simulink model "Scenario_TJunction_noTrafficLights_older"  (R2021a)
settings: Solver=VariableStepAuto  StartTime=0.0  StopTime=10.0  RelTol=1e-3
model workspace (MAT data in the model file):
  Kz_dif = Simulink.Parameter
  Kz_dif.Value = Simulink.data.Expression
  Kz_dif.Value.ExpressionString = " L_dif / (Lc + ds)"
  Kz_dif.DataType = 'auto'
  Kz_dif.Dimensions = -1
  Kz_il = Simulink.Parameter
  Kz_il.Value = Simulink.data.Expression
  Kz_il.Value.ExpressionString = " L_il / (Lc + ds)"
  Kz_il.DataType = 'auto'
  Kz_il.Dimensions = -1
  Kz_ir = Simulink.Parameter
  Kz_ir.Value = Simulink.data.Expression
  Kz_ir.Value.ExpressionString = " L_ir / (Lc + ds)"
  Kz_ir.DataType = 'auto'
  Kz_ir.Dimensions = -1
  Kz_is = Simulink.Parameter
  Kz_is.Value = Simulink.data.Expression
  Kz_is.Value.ExpressionString = " L_is / (Lc + ds)"
  Kz_is.DataType = 'auto'
  Kz_is.Dimensions = -1
  Kz_long = Simulink.Parameter
  Kz_long.Value = Simulink.data.Expression
  Kz_long.Value.ExpressionString = " L_long / (Lc + ds)"
  Kz_long.Description = 'Segmentkapazität (wie viele autos passen hinein)'
  Kz_long.DataType = 'auto'
  Kz_long.Dimensions = -1
  Kz_pre = Simulink.Parameter
  Kz_pre.Value = Simulink.data.Expression
  Kz_pre.Value.ExpressionString = " L_pre / (Lc + ds)"
  Kz_pre.DataType = 'auto'
  Kz_pre.Dimensions = -1
  L_dif = Simulink.Parameter
  L_dif.Value = Simulink.data.Expression
  L_dif.Value.ExpressionString = "L_long-L_pre"
  L_dif.Description = 'Differenz zwischen Abbiegerspurlänge und normaler straßenlänge'
  L_dif.DataType = 'auto'
  L_dif.Dimensions = -1
  L_il = Simulink.Parameter
  L_il.Value = 30
  L_il.Description = 'Länge der innenkreuzungssegments, das linksabbieger durchqueren'
  L_il.DataType = 'auto'
  L_il.Dimensions = [1 1]
  L_ir = Simulink.Parameter
  L_ir.Value = 23
  L_ir.Description = 'Länge der innenkreuzungssegments, das rechtsabbieger durchqueren'
  L_ir.DataType = 'auto'
  L_ir.Dimensions = [1 1]
  L_is = Simulink.Parameter
  L_is.Value = 35
  L_is.Description = 'Länge der innenkreuzungssegments, das geradeausfahrer durchqueren'
  L_is.DataType = 'auto'
  L_is.Dimensions = [1 1]
  L_long = Simulink.Parameter
  L_long.Value = 52.8
  L_long.Description = 'Langes straßensegment  (52.8 meter)'
  L_long.DataType = 'auto'
  L_long.Dimensions = [1 1]
  L_pre = Simulink.Parameter
  L_pre.Value = 20
  L_pre.Description = 'Länge der Abbiegespuren'
  L_pre.DataType = 'auto'
  L_pre.Dimensions = [1 1]
  Lc = Simulink.Parameter
  Lc.Value = 4.4
  Lc.Description = 'Länge eines autos'
  Lc.DataType = 'auto'
  Lc.Dimensions = [1 1]
  Rk = Simulink.Parameter
  Rk.Value = Simulink.data.Expression
  Rk.Value.ExpressionString = " Lc / v"
  Rk.Description = 'Flussrate zwischen den Kanten (bei speed v)'
  Rk.DataType = 'auto'
  Rk.Dimensions = -1
  Tz_dif = Simulink.Parameter
  Tz_dif.Value = Simulink.data.Expression
  Tz_dif.Value.ExpressionString = " L_dif / v"
  Tz_dif.DataType = 'auto'
  Tz_dif.Dimensions = -1
  Tz_il = Simulink.Parameter
  Tz_il.Value = Simulink.data.Expression
  Tz_il.Value.ExpressionString = " L_il / v"
  Tz_il.DataType = 'auto'
  Tz_il.Dimensions = -1
  Tz_ir = Simulink.Parameter
  Tz_ir.Value = Simulink.data.Expression
  Tz_ir.Value.ExpressionString = " L_ir / v"
  Tz_ir.DataType = 'auto'
  Tz_ir.Dimensions = -1
  Tz_is = Simulink.Parameter
  Tz_is.Value = Simulink.data.Expression
  Tz_is.Value.ExpressionString = " L_is / v"
  Tz_is.DataType = 'auto'
  Tz_is.Dimensions = -1
  Tz_long = Simulink.Parameter
  Tz_long.Value = Simulink.data.Expression
  Tz_long.Value.ExpressionString = " L_long / v"
  Tz_long.Description = 'Segment durchfahrtzeit: wie lange würde ein auto brauchen,um
    | ungehindert durch das segment zu fahren.'
  Tz_long.DataType = 'auto'
  Tz_long.Dimensions = -1
  Tz_pre = Simulink.Parameter
  Tz_pre.Value = Simulink.data.Expression
  Tz_pre.Value.ExpressionString = " L_pre / v"
  Tz_pre.DataType = 'auto'
  Tz_pre.Dimensions = -1
  ds = Simulink.Parameter
  ds.Value = Simulink.data.Expression
  ds.Value.ExpressionString = "v*dt"
  ds.DataType = 'auto'
  ds.Dimensions = -1
  dt = Simulink.Parameter
  dt.Value = 1
  dt.Description = 'temporaler sicherheitsabstand'
  dt.DataType = 'auto'
  dt.Dimensions = [1 1]
  v = Simulink.Parameter
  v.Value = 13.89
  v.Description = 'geschwindigkeit eines autos
    | (km/h : 3.75 = m/s)
    | 	30km/h = 8,34m/s
    | 	20km/h = 5.56m/s
    | 	50km/h = 13.89m/s
    | '
  v.DataType = 'auto'
  v.Dimensions = [1 1]
libraries: EdgesLibrary x26, StreetLanesLibrary x24, SourcesAndSinksLibrary x6
settings Model: Creator=phill  LastModifiedBy=phill
settings SolverCC: ZeroCrossAlgorithm=Adaptive

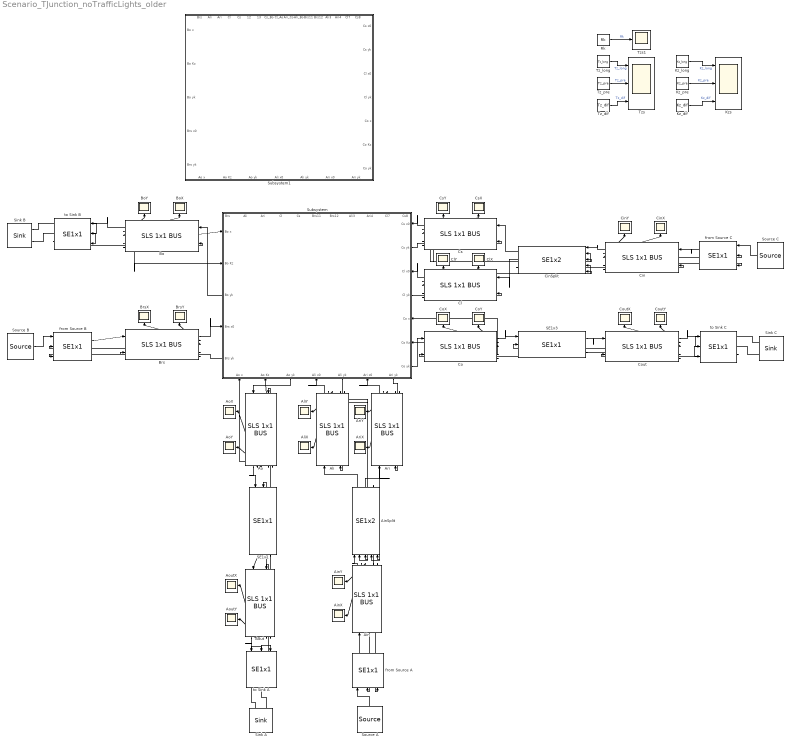
== system Scenario_TJunction_noTrafficLights_older ==
  Ain : StreetLanesLibrary/SLS 1x1 BUS  Kz=Kz_dif  Tz=Tz_dif
  AinSplit : EdgesLibrary/SE1x2  Rk1=0.5*Rk  Rk2=0.5*Rk
  AinX : Scope
  AinY : Scope
  Ali : StreetLanesLibrary/SLS 1x1 BUS  Kz=Kz_pre  Tz=Tz_pre
  AliX : Scope
  AliY : Scope
  Ao : StreetLanesLibrary/SLS 1x1 BUS  Kz=Kz_pre  Tz=Tz_pre
  AoX : Scope
  AoY : Scope
  Aout : StreetLanesLibrary/SLS 1x1 BUS  Kz=Kz_dif  Tz=Tz_dif
  AoutX : Scope
  AoutY : Scope
  Ari : StreetLanesLibrary/SLS 1x1 BUS  Kz=Kz_pre  Tz=Tz_pre
  AriX : Scope
  AriY : Scope
  Bo : StreetLanesLibrary/SLS 1x1 BUS  Kz=Kz_pre  Tz=Tz_pre
  BoX : Scope
  BoY : Scope
  Brs : StreetLanesLibrary/SLS 1x1 BUS  Kz=Kz_pre  Tz=Tz_pre
  BrsX : Scope
  BrsY : Scope
  Cin : StreetLanesLibrary/SLS 1x1 BUS  Kz=Kz_dif  Tz=Tz_dif
  CinSplit : EdgesLibrary/SE1x2  Rk1=0.5*Rk  Rk2=0.5*Rk
  CinX : Scope
  CinY : Scope
  Cl : StreetLanesLibrary/SLS 1x1 BUS  Kz=Kz_pre  Tz=Tz_pre
  ClX : Scope
  ClY : Scope
  Co : StreetLanesLibrary/SLS 1x1 BUS  Kz=Kz_pre  Tz=Tz_pre
  CoX : Scope
  CoY : Scope
  Cout : StreetLanesLibrary/SLS 1x1 BUS  Kz=Kz_dif  Tz=Tz_dif
  CoutX : Scope
  CoutY : Scope
  Cs : StreetLanesLibrary/SLS 1x1 BUS  Kz=Kz_pre  Tz=Tz_pre
  CsX : Scope
  CsY : Scope
  Kz_dif : Constant  Value=Kz_dif
  Kz_long : Constant  Value=Kz_long
  Kz_pre : Constant  Value=Kz_pre
  Kzs : Scope  NumInputPorts=3
  Rk : Constant  Value=Rk
  SE1x1 : EdgesLibrary/SE1x1  Rk=Rk
  SE1x3 : EdgesLibrary/SE1x1  Rk=Rk
  Sink A : SourcesAndSinksLibrary/Sink  SystemSampleTime=-1  VariantActivationTime=update diagram  Latency=0  AutoFrameSizeCalculation=off
      settings: PortSchema="{\"entries\":[{\"content\":{\"sides\":[{\"content\":{\"connectorIds\":[\"Out1\",\"Out2\"]},\"type\":\"ConnectorPlacement.EquallySpacedRectSide\",\"uuid\":\"9fd2383e-3590-4f0f-bafc-5a4adfbb32b4\"},{\"content\":{\"connectorIds\":[],\"side\":\"RIGHT\"},\"type\":\"ConnectorPlacement.EquallySpacedRectSide\",\"uuid\":\"1e687aa9-1098-45bd-a1f6-ea403f3f2897\"},{\"content\":{\"connectorIds\":[],\"side\":\"TOP\"},\"type\":\"ConnectorPlacement.EquallySpacedRectSide\",\"uuid\":\"fe6eaa71-085c-414b-983a-a0e72e52a49c\"}]},\"type\":\"ConnectorPlacement.EquallySpacedConnector\",\"uuid\":\"370c1712-4373-4726-99c2-6cb04807ece1\"}],\"packageUris\":[\"http://schema.mathworks.com/mf0/Connector/R2020b\"],\"version\":\"1.0\"}"
  Sink B : SourcesAndSinksLibrary/Sink  SystemSampleTime=-1  VariantActivationTime=update diagram  Latency=0  AutoFrameSizeCalculation=off
      settings: PortSchema="{\"entries\":[{\"content\":{\"sides\":[{\"content\":{\"connectorIds\":[\"Out1\",\"Out2\"]},\"type\":\"ConnectorPlacement.EquallySpacedRectSide\",\"uuid\":\"9fd2383e-3590-4f0f-bafc-5a4adfbb32b4\"},{\"content\":{\"connectorIds\":[],\"side\":\"RIGHT\"},\"type\":\"ConnectorPlacement.EquallySpacedRectSide\",\"uuid\":\"1e687aa9-1098-45bd-a1f6-ea403f3f2897\"},{\"content\":{\"connectorIds\":[],\"side\":\"TOP\"},\"type\":\"ConnectorPlacement.EquallySpacedRectSide\",\"uuid\":\"fe6eaa71-085c-414b-983a-a0e72e52a49c\"}]},\"type\":\"ConnectorPlacement.EquallySpacedConnector\",\"uuid\":\"370c1712-4373-4726-99c2-6cb04807ece1\"}],\"packageUris\":[\"http://schema.mathworks.com/mf0/Connector/R2020b\"],\"version\":\"1.0\"}"
  Sink C : SourcesAndSinksLibrary/Sink  SystemSampleTime=-1  VariantActivationTime=update diagram  Latency=0  AutoFrameSizeCalculation=off
      settings: PortSchema="{\"entries\":[{\"content\":{\"sides\":[{\"content\":{\"connectorIds\":[\"Out1\",\"Out2\"]},\"type\":\"ConnectorPlacement.EquallySpacedRectSide\",\"uuid\":\"9fd2383e-3590-4f0f-bafc-5a4adfbb32b4\"},{\"content\":{\"connectorIds\":[],\"side\":\"RIGHT\"},\"type\":\"ConnectorPlacement.EquallySpacedRectSide\",\"uuid\":\"1e687aa9-1098-45bd-a1f6-ea403f3f2897\"},{\"content\":{\"connectorIds\":[],\"side\":\"TOP\"},\"type\":\"ConnectorPlacement.EquallySpacedRectSide\",\"uuid\":\"fe6eaa71-085c-414b-983a-a0e72e52a49c\"}]},\"type\":\"ConnectorPlacement.EquallySpacedConnector\",\"uuid\":\"370c1712-4373-4726-99c2-6cb04807ece1\"}],\"packageUris\":[\"http://schema.mathworks.com/mf0/Connector/R2020b\"],\"version\":\"1.0\"}"
  Source A : SourcesAndSinksLibrary/Source  SystemSampleTime=-1  VariantActivationTime=update diagram  Latency=0  AutoFrameSizeCalculation=off
  Source B : SourcesAndSinksLibrary/Source  SystemSampleTime=-1  VariantActivationTime=update diagram  Latency=0  AutoFrameSizeCalculation=off
  Source C : SourcesAndSinksLibrary/Source  SystemSampleTime=-1  VariantActivationTime=update diagram  Latency=0  AutoFrameSizeCalculation=off
  Subsystem : Subsystem  mask{Kz_left=Kz_il, Tz_left=Tz_il, Kz_straight=Kz_is, Tz_straight=Tz_is, Kz_right=Kz_ir, Tz_right=Tz_ir, Rk=Rk}
      settings: PortSchema="{\"entries\":[{\"content\":{\"sides\":[{\"content\":{\"connectorIds\":[\"In1\",\"In2\",\"Out12\",\"In3\",\"Out13\"]},\"type\":\"ConnectorPlacement.EquallySpacedRectSide\",\"uuid\":\"e697a1b6-0b61-4022-ac11-26e96db57f42\"},{\"content\":{\"connectorIds\":[\"In14\",\"Out1\",\"In15\",\"Out2\",\"In16\",\"In17\",\"Out3\"],\"side\":\"RIGHT\"},\"type\":\"ConnectorPlacement.EquallySpacedRectSide\",\"uuid\":\"73d64b2d-08c1-4421-9fcb-daf7d69c3a51\"},{\"content\":{\"connectorIds\":[\"Out7\",\"Out8\",\"Out9\",\"Out10\",\"Out11\",\"In4\",\"In5\",\"In6\",\"In7\",\"In8\",\"In9\"],\"side\":\"TOP\"},\"type\":\"ConnectorPlacement.EquallySpacedRectSide\",\"uuid\":\"d1fda098-bb61-48fd-b619-252fd8b1727b\"},{\"content\":{\"connectorIds\":[\"In10\",\"In11\",\"Out4\",\"In12\",\"Out5\",\"In13\",\"Out6\"],\"side\":\"BOTTOM\"},\"type\":\"ConnectorPlacement.EquallySpacedRectSide\",\"uuid\":\"eb83420e-ae17-428e-89d3-8e583c14dd5f\"}]},\"type\":\"ConnectorPlacement.EquallySpacedConnector\",\"uuid\":\"f702b239-8bcf-4357-be27-0d0ceba5c268\"}],\"packageUris\":[\"http://schema.mathworks.com/mf0/Connector/R2020b\"],\"version\":\"1.0\"}"
      mask Display:
      | %image('$imagefile'); % Use "Edit Image" on toolstrip to change.
      | disp('T \n\n');
      | KzS = get_param(gcb,'Kz_straight');
      | TzS = get_param(gcb,'Tz_straight');
      | KzR = get_param(gcb,'Kz_right');
      | TzR = get_param(gcb,'Tz_right');
      | KzL = get_param(gcb,'Kz_left');
      | TzL = get_param(gcb,'Tz_left');
      | Rk = get_param(gcb,'Rk');
      | disp(['Rk = ', Rk, ' | Kz/Tz L = ', KzL, ' ', TzL, ' | Kz/Tz S = ', KzS, ' ', TzS, ' | Kz/Tz R = ', KzR, ' ', TzR]);
  Subsystem1 : Subsystem  mask{Kz_left=0, Tz_left=0, Kz_straight=0, Tz_straight=0, Kz_right=0, Tz_right=0, Rk=0}
      settings: PortSchema="{\"entries\":[{\"content\":{\"sides\":[{\"content\":{\"connectorIds\":[\"In1\",\"In2\",\"Out18\",\"In3\",\"Out19\"]},\"type\":\"ConnectorPlacement.EquallySpacedRectSide\",\"uuid\":\"96c9f498-b0bc-4839-a476-8992d885d35a\"},{\"content\":{\"connectorIds\":[\"In14\",\"Out1\",\"In15\",\"Out2\",\"In16\",\"In17\",\"Out3\"],\"side\":\"RIGHT\"},\"type\":\"ConnectorPlacement.EquallySpacedRectSide\",\"uuid\":\"11ab0cdd-7db6-4f39-a252-8216aa6322d2\"},{\"content\":{\"connectorIds\":[\"Out7\",\"Out8\",\"Out9\",\"Out10\",\"Out11\",\"Out12\",\"Out13\",\"Out14\",\"Out15\",\"Out16\",\"Out17\",\"In4\",\"In5\",\"In6\",\"In7\",\"In8\",\"In9\"],\"side\":\"TOP\"},\"type\":\"ConnectorPlacement.EquallySpacedRectSide\",\"uuid\":\"f8ff7b80-df82-4633-b83a-80e44c4409b9\"},{\"content\":{\"connectorIds\":[\"In10\",\"In11\",\"Out4\",\"In12\",\"Out5\",\"In13\",\"Out6\"],\"side\":\"BOTTOM\"},\"type\":\"ConnectorPlacement.EquallySpacedRectSide\",\"uuid\":\"816219a6-152c-447e-807e-ad4d62c96b47\"}]},\"type\":\"ConnectorPlacement.EquallySpacedConnector\",\"uuid\":\"16c591aa-9a6b-4cb9-9c60-a78ca06e8a6b\"}],\"packageUris\":[\"http://schema.mathworks.com/mf0/Connector/R2020b\"],\"version\":\"1.0\"}"
      mask Display:
      | %image('$imagefile'); % Use "Edit Image" on toolstrip to change.
      | disp('T \n\n');
      | KzS = get_param(gcb,'Kz_straight');
      | TzS = get_param(gcb,'Tz_straight');
      | KzR = get_param(gcb,'Kz_right');
      | TzR = get_param(gcb,'Tz_right');
      | KzL = get_param(gcb,'Kz_left');
      | TzL = get_param(gcb,'Tz_left');
      | Rk = get_param(gcb,'Rk');
      | disp(['Rk = ', Rk, ' | Kz/Tz L = ', KzL, ' ', TzL, ' | Kz/Tz S = ', KzS, ' ', TzS, ' | Kz/Tz R = ', KzR, ' ', TzR]);
  Tz_dif : Constant  Value=Tz_dif
  Tz_long : Constant  Value=Tz_long
  Tz_pre : Constant  Value=Tz_pre
  Tzs : Scope  NumInputPorts=3
  Tzs1 : Scope
  from Source A : EdgesLibrary/SE1x1  Rk=Rk
  from Source B : EdgesLibrary/SE1x1  Rk=Rk
  from Source C : EdgesLibrary/SE1x1  Rk=Rk
  to Sink A : EdgesLibrary/SE1x1  Rk=Rk
  to Sink B : EdgesLibrary/SE1x1  Rk=Rk
  to Sink C : EdgesLibrary/SE1x1  Rk=Rk
  wires:
  Ao/6 -> Subsystem/10(Ao x)
  Ao/7 -> Subsystem/11(Ao Kz)
  Subsystem/4(Ao yk) -> Ao/1
  Ali/2 -> Subsystem/12(Ali x0)
  Subsystem/5(Ali yk) -> Ali/2
  Ari/2 -> Subsystem/13(Ari x0)
  Subsystem/6(Ari yk) -> Ari/2
  AinSplit/2 -> Ari/1
  Ari/7 -> AinSplit/5
  Ari/6 -> AinSplit/4
  AinSplit/1 -> Ali/1
  Ali/7 -> AinSplit/3
  Ali/6 -> AinSplit/2
  Ao/2 -> SE1x1/1
  SE1x1/2 -> Ao/2
  Ain/2 -> AinSplit/1
  AinSplit/3 -> Ain/2
  Aout/6 -> SE1x1/2
  Aout/7 -> SE1x1/3
  SE1x1/1 -> Aout/1
  Source A/1 -> from Source A/1
  from Source A/1 -> Ain/1
  Ain/7 -> from Source A/3
  Ain/6 -> from Source A/2
  to Sink A/2 -> Aout/2
  Aout/2 -> to Sink A/1
  Sink A/1 -> to Sink A/2
  Sink A/2 -> to Sink A/3
  Co/6 -> Subsystem/16(Co x)
  Co/7 -> Subsystem/17(Co Kz)
  Subsystem/3(Co yk) -> Co/1
  Subsystem/2(Cl yk) -> Cl/2
  Cl/2 -> Subsystem/15(Cl x0)
  Subsystem/1(Cs yk) -> Cs/2
  Cs/2 -> Subsystem/14(Cs x0)
  Bo/6 -> Subsystem/1(Bo x)
  Bo/7 -> Subsystem/2(Bo Kz)
  Subsystem/12(Bo yk) -> Bo/1
  Brs/2 -> Subsystem/3(Brs x0)
  Subsystem/13(Brs yk) -> Brs/2
  SE1x3/2 -> Co/2
  Co/2 -> SE1x3/1
  SE1x3/1 -> Cout/1
  Cout/7 -> SE1x3/3
  Cout/6 -> SE1x3/2
  Cs/6 -> CinSplit/2
  Cs/7 -> CinSplit/3
  CinSplit/1 -> Cs/1
  Cl/6 -> CinSplit/4
  Cl/7 -> CinSplit/5
  CinSplit/2 -> Cl/1
  CinSplit/3 -> Cin/2
  Cin/2 -> CinSplit/1
  Sink C/1 -> to Sink C/2
  Sink C/2 -> to Sink C/3
  Cout/2 -> to Sink C/1
  to Sink C/2 -> Cout/2
  Source C/1 -> from Source C/1
  Cin/6 -> from Source C/2
  Cin/7 -> from Source C/3
  from Source C/1 -> Cin/1
  Source B/1 -> from Source B/1
  Sink B/2 -> to Sink B/3
  Sink B/1 -> to Sink B/2
  Bo/2 -> to Sink B/1
  to Sink B/2 -> Bo/2
  Brs/6 -> from Source B/2
  Brs/7 -> from Source B/3
  from Source B/1 -> Brs/1
  Bo/4 -> BoY/1
  Cs/4 -> CsY/1
  Cl/4 -> ClY/1
  Cl/3 -> ClX/1
  Co/3 -> CoX/1
  Co/4 -> CoY/1
  Cs/3 -> CsX/1
  Brs/3 -> BrsX/1
  Brs/4 -> BrsY/1
  Bo/3 -> BoX/1
  Cin/4 -> CinY/1
  Cin/3 -> CinX/1
  Cout/3 -> CoutX/1
  Cout/4 -> CoutY/1
  Ao/3 -> AoX/1
  Ao/4 -> AoY/1
  Ali/4 -> AliY/1
  Ali/3 -> AliX/1
  Ari/4 -> AriY/1
  Ari/3 -> AriX/1
  Aout/3 -> AoutX/1
  Aout/4 -> AoutY/1
  Ain/4 -> AinY/1
  Ain/3 -> AinX/1
  Tz_long/1 -> Tzs/1  "Tz_long"
  Tz_pre/1 -> Tzs/2  "Tz_pre"
  Tz_dif/1 -> Tzs/3  "Tz_dif"
  Kz_long/1 -> Kzs/1  "Kz_long"
  Kz_pre/1 -> Kzs/2  "Kz_pre"
  Kz_dif/1 -> Kzs/3  "Kz_dif"
  Rk/1 -> Tzs1/1  "Rk"

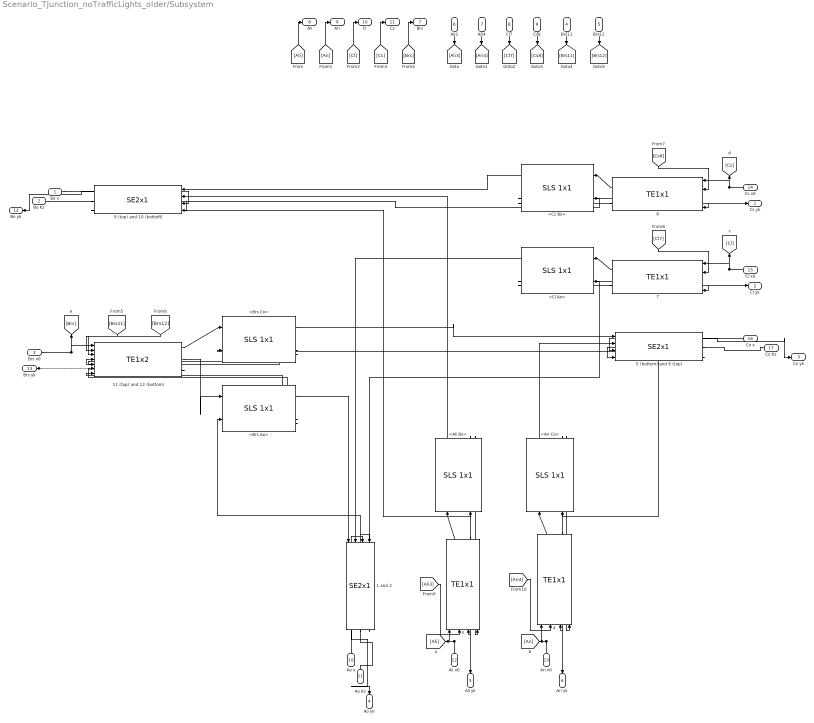
== system Scenario_TJunction_noTrafficLights_older/Subsystem ==
  Bo x : Inport
  Bo Kz : Inport  Port=2
  Brs x0 : Inport  Port=3
  Brs11 : Inport  Port=4
  Brs12 : Inport  Port=5
  Ali3 : Inport  Port=6
  Ari4 : Inport  Port=7
  Cl7 : Inport  Port=8
  Cs8 : Inport  Port=9
  Ao x : Inport  Port=10
  Ao Kz : Inport  Port=11
  Ali x0 : Inport  Port=12
  Ari x0 : Inport  Port=13
  Cs x0 : Inport  Port=14
  Cl x0 : Inport  Port=15
  Co x : Inport  Port=16
  Co Kz : Inport  Port=17
  1 and 2 : EdgesLibrary/SE2x1  Rk1=Rk  Rk2=Rk
  11 (top) and 12 (bottom) : EdgesLibrary/TE1x2  Rk1=0.5*Rk  Rk2=0.5*Rk
  {3..4,7..8} (4 alike) : EdgesLibrary/TE1x1  Rk=Rk
  5 (bottom) and 6 (top) : EdgesLibrary/SE2x1  Rk1=Rk  Rk2=Rk
  9 (top) and 10 (bottoM) : EdgesLibrary/SE2x1  Rk1=Rk  Rk2=Rk
  <Ali Bo> : StreetLanesLibrary/SLS 1x1  Kz=Kz_left  Tz=Tz_left
  <Ari Co> : StreetLanesLibrary/SLS 1x1  Kz=Kz_right  Tz=Tz_right
  <Brs Ao> : StreetLanesLibrary/SLS 1x1  Kz=Kz_right  Tz=Tz_right
  <Brs Co> : StreetLanesLibrary/SLS 1x1  Kz=Kz_straight  Tz=Tz_straight
  <Cl Ao> : StreetLanesLibrary/SLS 1x1  Kz=Kz_left  Tz=Tz_left
  <Cs Bo> : StreetLanesLibrary/SLS 1x1  Kz=Kz_straight  Tz=Tz_straight
  Cs yk : Outport
  Cl yk : Outport  Port=2
  Co yk : Outport  Port=3
  Ao yk : Outport  Port=4
  Ali yk : Outport  Port=5
  Ari yk : Outport  Port=6
  Brs : Outport  Port=7
  Ali : Outport  Port=8
  Ari : Outport  Port=9
  Cl : Outport  Port=10
  Cs : Outport  Port=11
  Bo yk : Outport  Port=12
  Brs yk : Outport  Port=13
  wires:
  11 (top) and 12 (bottom)/2 -> <Brs Ao>/1
  11 (top) and 12 (bottom)/3 -> Brs yk/1
  3/2 -> Ali yk/1
  3/1 -> <Ali Bo>/1
  Ari x0/1 -> [Ari], 4/1
  <Cs Bo>/2 -> 9 (top) and 10 (bottoM)/1
  <Cs Bo>/8 -> 8/4
  <Cl Ao>/8 -> 7/4
  Co x/1 -> 5 (bottom) and 6 (top)/3
  5 (bottom) and 6 (top)/1 -> Co yk/1
  5 (bottom) and 6 (top)/3 -> <Ari Co>/2
  <Ari Co>/8 -> 4/4
  <Ali Bo>/8 -> 3/4
  Ao x/1 -> 1 and 2/3
  Brs x0/1 -> 11 (top) and 12 (bottom)/1, [Brs]
  <Brs Co>/2 -> 5 (bottom) and 6 (top)/1
  <Cl Ao>/7 -> 7/3
  <Cl Ao>/2 -> 1 and 2/2
  9 (top) and 10 (bottoM)/2 -> <Cs Bo>/2
  [Brs] -> Brs/1
  <Ari Co>/2 -> 5 (bottom) and 6 (top)/2
  7/1 -> <Cl Ao>/1
  Cl x0/1 -> [Cl], 7/1
  4/1 -> <Ari Co>/1
  <Ari Co>/7 -> 4/3
  <Brs Ao>/2 -> 1 and 2/1
  Ao Kz/1 -> 1 and 2/4
  <Brs Ao>/7 -> 11 (top) and 12 (bottom)/6
  <Brs Ao>/8 -> 11 (top) and 12 (bottom)/7
  Co Kz/1 -> 5 (bottom) and 6 (top)/4
  8/2 -> Cs yk/1
  Bo Kz/1 -> 9 (top) and 10 (bottoM)/4
  1 and 2/3 -> <Cl Ao>/2
  <Brs Co>/8 -> 11 (top) and 12 (bottom)/5
  [Brs12] -> 11 (top) and 12 (bottom)/3
  9 (top) and 10 (bottoM)/3 -> <Ali Bo>/2
  <Ali Bo>/7 -> 3/3
  1 and 2/2 -> <Brs Ao>/2
  Ali x0/1 -> [Ali], 3/1
  <Brs Co>/7 -> 11 (top) and 12 (bottom)/4
  1 and 2/1 -> Ao yk/1
  <Ali Bo>/2 -> 9 (top) and 10 (bottoM)/2
  [Ari4] -> 4/2
  5 (bottom) and 6 (top)/2 -> <Brs Co>/2
  8/1 -> <Cs Bo>/1
  4/2 -> Ari yk/1
  <Cs Bo>/7 -> 8/3
  Cs x0/1 -> [Cs], 8/1
  [Ali3] -> 3/2
  [Brs11] -> 11 (top) and 12 (bottom)/2
  11 (top) and 12 (bottom)/1 -> <Brs Co>/1
  Bo x/1 -> 9 (top) and 10 (bottoM)/3
  [Cl7] -> 7/2
  9 (top) and 10 (bottoM)/1 -> Bo yk/1
  [Ari] -> Ari/1
  [Ali] -> Ali/1
  7/2 -> Cl yk/1
  [Cs8] -> 8/2
  [Cl] -> Cl/1
  [Cs] -> Cs/1
  Ali3/1 -> [Ali3]
  Ari4/1 -> [Ari4]
  Cl7/1 -> [Cl7]
  Cs8/1 -> [Cs8]
  Brs11/1 -> [Brs11]
  Brs12/1 -> [Brs12]

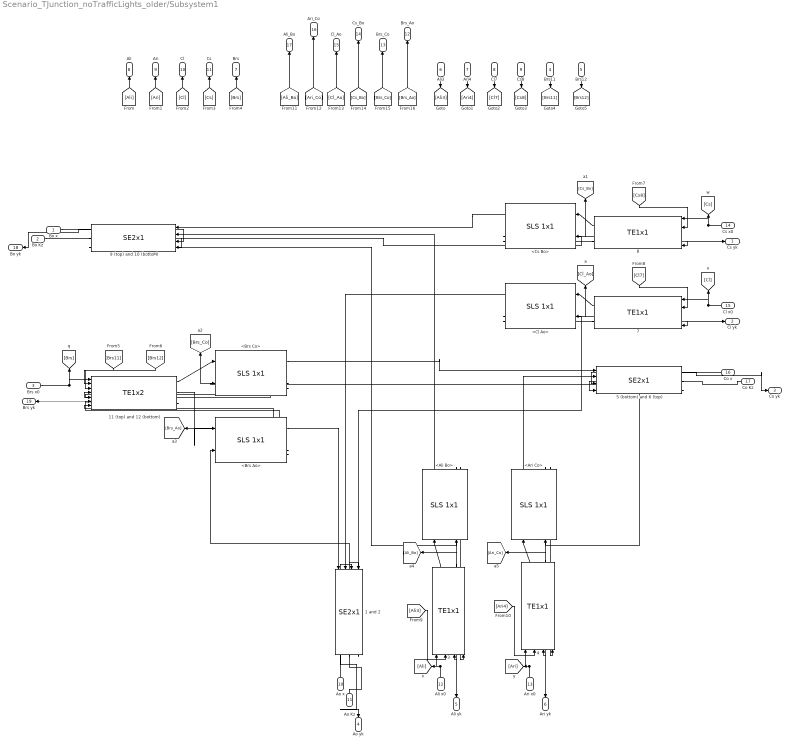
== system Scenario_TJunction_noTrafficLights_older/Subsystem1 ==
  Bo x : Inport
  Bo Kz : Inport  Port=2
  Brs x0 : Inport  Port=3
  Brs11 : Inport  Port=4
  Brs12 : Inport  Port=5
  Ali3 : Inport  Port=6
  Ari4 : Inport  Port=7
  Cl7 : Inport  Port=8
  Cs8 : Inport  Port=9
  Ao x : Inport  Port=10
  Ao Kz : Inport  Port=11
  Ali x0 : Inport  Port=12
  Ari x0 : Inport  Port=13
  Cs x0 : Inport  Port=14
  Cl x0 : Inport  Port=15
  Co x : Inport  Port=16
  Co Kz : Inport  Port=17
  1 and 2 : EdgesLibrary/SE2x1  Rk1=Rk  Rk2=Rk
  11 (top) and 12 (bottom) : EdgesLibrary/TE1x2  Rk1=0.5*Rk  Rk2=0.5*Rk
  {3..4,7..8} (4 alike) : EdgesLibrary/TE1x1  Rk=Rk
  5 (bottom) and 6 (top) : EdgesLibrary/SE2x1  Rk1=Rk  Rk2=Rk
  9 (top) and 10 (bottoM) : EdgesLibrary/SE2x1  Rk1=Rk  Rk2=Rk
  <Ali Bo> : StreetLanesLibrary/SLS 1x1  Kz=Kz_left  Tz=Tz_left
  <Ari Co> : StreetLanesLibrary/SLS 1x1  Kz=Kz_right  Tz=Tz_right
  <Brs Ao> : StreetLanesLibrary/SLS 1x1  Kz=Kz_right  Tz=Tz_right
  <Brs Co> : StreetLanesLibrary/SLS 1x1  Kz=Kz_straight  Tz=Tz_straight
  <Cl Ao> : StreetLanesLibrary/SLS 1x1  Kz=Kz_left  Tz=Tz_left
  <Cs Bo> : StreetLanesLibrary/SLS 1x1  Kz=Kz_straight  Tz=Tz_straight
  Cs yk : Outport
  Cl yk : Outport  Port=2
  Co yk : Outport  Port=3
  Ao yk : Outport  Port=4
  Ali yk : Outport  Port=5
  Ari yk : Outport  Port=6
  Brs : Outport  Port=7
  Ali : Outport  Port=8
  Ari : Outport  Port=9
  Cl : Outport  Port=10
  Cs : Outport  Port=11
  Brs_Ao : Outport  Port=12
  Brs_Co : Outport  Port=13
  Cs_Bo : Outport  Port=14
  Cl_Ao : Outport  Port=15
  Ari_Co : Outport  Port=16
  Ali_Bo : Outport  Port=17
  Bo yk : Outport  Port=18
  Brs yk : Outport  Port=19
  wires:
  11 (top) and 12 (bottom)/2 -> <Brs Ao>/1
  11 (top) and 12 (bottom)/3 -> Brs yk/1
  3/2 -> Ali yk/1
  3/1 -> <Ali Bo>/1
  Ari x0/1 -> [Ari], 4/1
  <Cs Bo>/2 -> 9 (top) and 10 (bottoM)/1
  <Cs Bo>/8 -> 8/4
  <Cl Ao>/8 -> 7/4
  Co x/1 -> 5 (bottom) and 6 (top)/3
  5 (bottom) and 6 (top)/1 -> Co yk/1
  5 (bottom) and 6 (top)/3 -> <Ari Co>/2
  <Ari Co>/8 -> 4/4
  <Ali Bo>/8 -> 3/4
  Ao x/1 -> 1 and 2/3
  Brs x0/1 -> 11 (top) and 12 (bottom)/1, [Brs]
  <Brs Co>/2 -> 5 (bottom) and 6 (top)/1
  <Cl Ao>/7 -> [Cl_Ao], 7/3
  <Cl Ao>/2 -> 1 and 2/2
  9 (top) and 10 (bottoM)/2 -> <Cs Bo>/2
  <Ari Co>/2 -> 5 (bottom) and 6 (top)/2
  7/1 -> <Cl Ao>/1
  Cl x0/1 -> [Cl], 7/1
  4/1 -> <Ari Co>/1
  <Ari Co>/7 -> 4/3, [Ari_Co]
  <Brs Ao>/2 -> 1 and 2/1
  Ao Kz/1 -> 1 and 2/4
  <Brs Ao>/7 -> [Brs_Ao], 11 (top) and 12 (bottom)/6
  <Brs Ao>/8 -> 11 (top) and 12 (bottom)/7
  Co Kz/1 -> 5 (bottom) and 6 (top)/4
  8/2 -> Cs yk/1
  Bo Kz/1 -> 9 (top) and 10 (bottoM)/4
  1 and 2/3 -> <Cl Ao>/2
  <Brs Co>/8 -> 11 (top) and 12 (bottom)/5
  [Brs12] -> 11 (top) and 12 (bottom)/3
  9 (top) and 10 (bottoM)/3 -> <Ali Bo>/2
  <Ali Bo>/7 -> 3/3, [Ali_Bo]
  1 and 2/2 -> <Brs Ao>/2
  Ali x0/1 -> [Ali], 3/1
  <Brs Co>/7 -> 11 (top) and 12 (bottom)/4, [Brs_Co]
  1 and 2/1 -> Ao yk/1
  <Ali Bo>/2 -> 9 (top) and 10 (bottoM)/2
  [Ari4] -> 4/2
  5 (bottom) and 6 (top)/2 -> <Brs Co>/2
  8/1 -> <Cs Bo>/1
  4/2 -> Ari yk/1
  <Cs Bo>/7 -> 8/3, [Cs_Bo]
  Cs x0/1 -> [Cs], 8/1
  [Ali3] -> 3/2
  [Brs11] -> 11 (top) and 12 (bottom)/2
  11 (top) and 12 (bottom)/1 -> <Brs Co>/1
  Bo x/1 -> 9 (top) and 10 (bottoM)/3
  [Cl7] -> 7/2
  9 (top) and 10 (bottoM)/1 -> Bo yk/1
  7/2 -> Cl yk/1
  [Cs8] -> 8/2
  [Ali_Bo] -> Ali_Bo/1
  [Ari_Co] -> Ari_Co/1
  [Cl_Ao] -> Cl_Ao/1
  [Cs_Bo] -> Cs_Bo/1
  [Brs_Co] -> Brs_Co/1
  [Brs_Ao] -> Brs_Ao/1
  [Ali] -> Ali/1
  [Ari] -> Ari/1
  [Cl] -> Cl/1
  [Cs] -> Cs/1
  [Brs] -> Brs/1
  Ali3/1 -> [Ali3]
  Ari4/1 -> [Ari4]
  Cl7/1 -> [Cl7]
  Cs8/1 -> [Cs8]
  Brs11/1 -> [Brs11]
  Brs12/1 -> [Brs12]
